simulink model "Stateflow_test"  (R2022a)
settings: Solver=FixedStepDiscrete  StartTime=0.0  StopTime=10.0  RelTol=1e-3  EnableMultiTasking=on
undefined symbols (not defined in the file): ESP, IDF, IP, TCP
libraries: esp32_io_lib x2, esp32_device_config_lib x1
settings Model: Creator=phank  LastModifiedBy=phank
settings SolverCC: PositivePriorityOrder=on  AutoInsertRateTranBlk=on
settings OptimizationCC: DefaultParameterBehavior=Inlined  EnhancedBackFolding=on  PassReuseOutputArgsAs=Individual arguments  ZeroExternalMemoryAtStartup=off  ZeroInternalMemoryAtStartup=off  OptimizeBlockOrder=speed  DifferentSizesBufferReuse=on  OptimizationCustomize=off  EfficientTunableParamExpr=on
settings DebuggingCC: ParameterTunabilityLossMsg=error
settings HardwareCC: ProdBitPerPointer=32  ProdBitPerSizeT=32  ProdBitPerPtrDiffT=32  ProdLargestAtomicInteger=Long  ProdLargestAtomicFloat=Double  ProdWordSize=32  ProdHWDeviceType=Cadence Design Systems (Tensilica)->Espressif Xtensa single-/dual-core 32-bit LX6 microprocessor
settings SFSimCC: MATLABDynamicMemAlloc=off
settings RTWCC: Description=Waijung 2 ESP32 target  SystemTargetFile=esp32.tlc  TemplateMakefile=esp32.tmf  RetainRTWFile=on
settings CodeAppCC: ForceParamTrailComments=on  IgnoreCustomStorageClasses=off  OperatorAnnotations=on  SimulinkDataObjDesc=on  SFDataObjDesc=on  InsertBlockDesc=on
settings STFCustomTargetCC: TargetLangStandard=C99 (ISO)  MultiwordLength=256  ModelReferenceCompliant=off  CombineOutputUpdateFcns=on  ERTCustomFileBanners=on  SupportContinuousTime=off  SupportNonInlinedSFcns=off  RemoveResetFunc=on  MATLABClassNameForMDSCustomization=Simulink.SoftwareTarget.ERTCustomization  GRTInterface=off  SystemTargetFile=esp32.tlc
settings ERTTargetCC: TargetLangStandard=C99 (ISO)  ModelReferenceCompliant=off  ParMdlRefBuildCompliant=off  CompOptLevelCompliant=off  ConcurrentExecutionCompliant=off  ModelStepFunctionPrototypeControlCompliant=off  CPPClassGenCompliant=off  UseToolchainInfoCompliant=off  ExtModeStaticAlloc=on  ExtModeStaticAllocSize=2048  InlinedParameterPlacement=NonHierarchical  ERTSrcFileBannerTemplate=esp32_code_template.cgt  ERTHdrFileBannerTemplate=esp32_code_template.cgt  ERTDataSrcFileTemplate=esp32_code_template.cgt  ERTDataHdrFileTemplate=esp32_code_template.cgt  ERTCustomFileTemplate=esp32_file_process.tlc

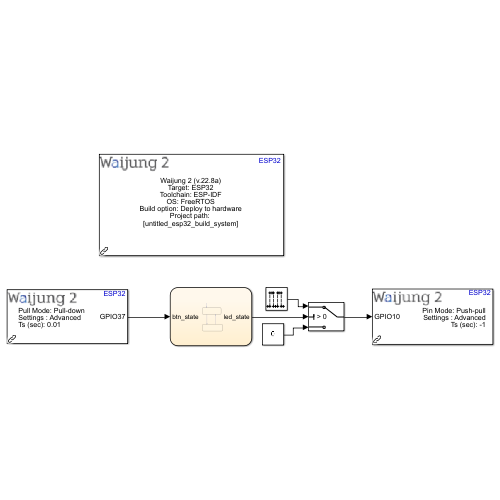
[thumbnail: Simulink's stored preview of the top-level diagram]
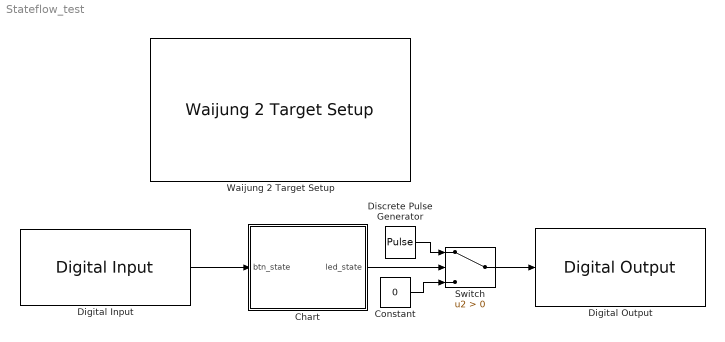
== system Stateflow_test ==
  Chart : Stateflow chart  TreatAsAtomicUnit=on
  Constant : Constant  Value=0  SampleTime=-1
  Digital Input : esp32_io_lib/Digital Input  blockid=DigitalInput  settings=Advanced  overridepin=off  pin0=off  pin1=off  pin2=off  pin3=off  pin4=off  pin5=off  pin6=off  pin7=off  pin8=off  pin9=off  pin10=off  pin11=off  pin12=off  pin13=off  pin14=off  pin15=off  pin16=off  pin17=off  pin18=off  pin19=off  pin20=off  pin21=off  pin22=off  pin23=off  pin24=off  pin25=off  pin26=off  pin27=off  pin28=off  pin29=off  pin30=off  pin31=off  pin32=off  pin33=off  pin34=off  pin35=off  pin36=off  pin37=on  pin38=off  pin39=off  pin40=off  pin41=off  pin42=off  pin43=off  pin44=off  pin45=off  pin46=off  pin47=off  pin48=off  pull_mode=Pull-down  pin_hold=Disable  deep_sleep_pin_hold=Disable  pin_array="[0  0  0  0  0  0  0  0  0  0  0  0  0  0  0  0  0  0  0  0  0  0  0  0  0  0  0  0  0  0  0  0  0  0  0  0  0  1  0  0  0  0  0  0  0  0  0  0  0]"  inport_num=1  pin_hold_define=off  pull_mode_define=GPIO_FLOATING  deep_sleep_pin_hold_define=off  pin_string=((1ULL<<37))  numpins=49  sampletime=0.01
      settings: SourceProductName=Waijung 2 Blockset
  Digital Output : esp32_io_lib/Digital Output  blockid=DigitalOutput  settings=Advanced  overridepin=on  pin0=off  pin1=off  pin2=off  pin3=off  pin4=off  pin5=off  pin6=off  pin7=off  pin8=off  pin9=off  pin10=on  pin11=off  pin12=off  pin13=off  pin14=off  pin15=off  pin16=off  pin17=off  pin18=off  pin19=off  pin20=off  pin21=off  pin22=off  pin23=off  pin24=off  pin25=off  pin26=off  pin27=off  pin28=off  pin29=off  pin30=off  pin31=off  pin32=off  pin33=off  pin34=off  pin35=off  pin36=off  pin37=off  pin38=off  pin39=off  pin40=off  pin41=off  pin42=off  pin43=off  pin44=off  pin45=off  pin46=off  pin47=off  pin48=off  pin_initialize=on  pin_mode=Push-pull  sampletime=-1  drive_capability=Normal (default)  pin_hold=Disable  deep_sleep_pin_hold=Disable  pin_array="[0  0  0  0  0  0  0  0  0  0  1  0  0  0  0  0  0  0  0  0  0  0  0  0  0  0  0  0  0  0  0  0  0  0  0  0  0  0  0  0  0  0  0  0  0  0  0  0  0]"  inport_num=1  drive_capability_define=GPIO_DRIVE_CAP_2  pin_hold_define=off  pin_mode_define=GPIO_MODE_INPUT_OUTPUT  deep_sleep_pin_hold_define=off  pin_string=((1ULL<<10))  numpins=49
      settings: SourceProductName=Waijung 2 Blockset
  Discrete Pulse Generator : DiscretePulseGenerator  Period=50  PulseWidth=25  SampleTime=0.01
  Switch : Switch  Criteria=u2 > Threshold  SaturateOnIntegerOverflow=off  InputSameDT=off
  Waijung 2 Target Setup : esp32_device_config_lib/Waijung 2 Target Setup  waijungversion=22.8a  toolchain=ESP-IDF  os=FreeRTOS  sampletime=-1  simulink_managebuildsystem=on  projectpath=untitled_esp32_build_system  espidfpath=C:\msys32\home\skris\esp\esp-idf  buildoptions=Deploy to hardware  blockid=Waijung2TargetSetup  target=ESP32  defaultstacksize=2048  basepriority=0  highestpriority=10  generate_baserate_task=on  tickrate=1000  esp32target=ESP32  esp32targetdef=esp32  esp32flashsize=4MB  esp32comport=<empty>  esp32baudrate=460800  esp32advancedconfig=off  esp32partitiontable=Use default waijung2 partition table  esp32partitionpath=Browse the partition table  partitionname=partitions.csv  editpartition=off  custompartitiondata={'nvs','data','nvs','','0x6000','';'phy_init','data','phy','','0x1000','';'factory','app','factory','','1M',''}  reqblocks=default  esp32custompartition={'nvs','data','nvs','','0x6000','';'phy_init','data','phy','','0x1000','';'factory','app','factory','','1M',''}  cominterface=TCP/IP  wifimode=WIFI AP  wifissid=esp32ssid  wifipassword=password  deviceip=192.168.1.10  targetgateway=192.168.1.1  targetnetmask=255.255.255.0  manualdns=on  targetdnsip=8.8.8.8  targetipport=256  targetipdef=0  targetmaskdef=0  targetgatewaydef=0  targetdnsipdef=0  hosttimeout=10  hostverbose=off
      settings: SourceProductName=Waijung 2 Blockset
  wires:
  Digital Input/1 -> Chart/1(btn_state)
  Discrete Pulse Generator/1 -> Switch/1
  Constant/1 -> Switch/3
  Chart/1(led_state) -> Switch/2
  Switch/1 -> Digital Output/1

== stateflow chart Stateflow_test/Chart ==
  state pattern1
    entry: led_state=0;
  state pattern2
    entry: led_state = 1;
  (default) -> pattern1
  pattern1 -> pattern2 : [btn_state == 0 && after(1,sec)]
  pattern2 -> pattern1 : [btn_state == 0 && after(1,sec)]
  data: btn_state input; led_state output
